simulink model "mesaparasimulink2"  (R2017a)
settings: Solver=ode3  StartTime=0.0  StopTime=3*1.256637  FixedStep=5e-3  RelTol=1e-3
values from neighbouring files (symbols this model uses):
  L1 = L1s(L1i)    [Resolver.m]    (also in calculodepar.m = L1/100)
  L2 = L2s(L2k)    [Resolver.m]    (also in calculodepar.m = L2/100)
  m = 6    [calculodepar.m]
  N = m*g - ten*sin(beta)    [calculodepar.m]    (also in main.m = 360; maindinamica.m = 360)
undefined symbols (not defined in the file or in its folder): bloque, bloque1, mesaparasimulink, pasador, RootGround, RootPart
libraries: mblibv1 x26, simulink x2
settings Model: Creator=angel  LastModifiedBy=angel
settings SimMechanicsCC: VisOnUpdateDiagram=on  VisDuringSimulation=on

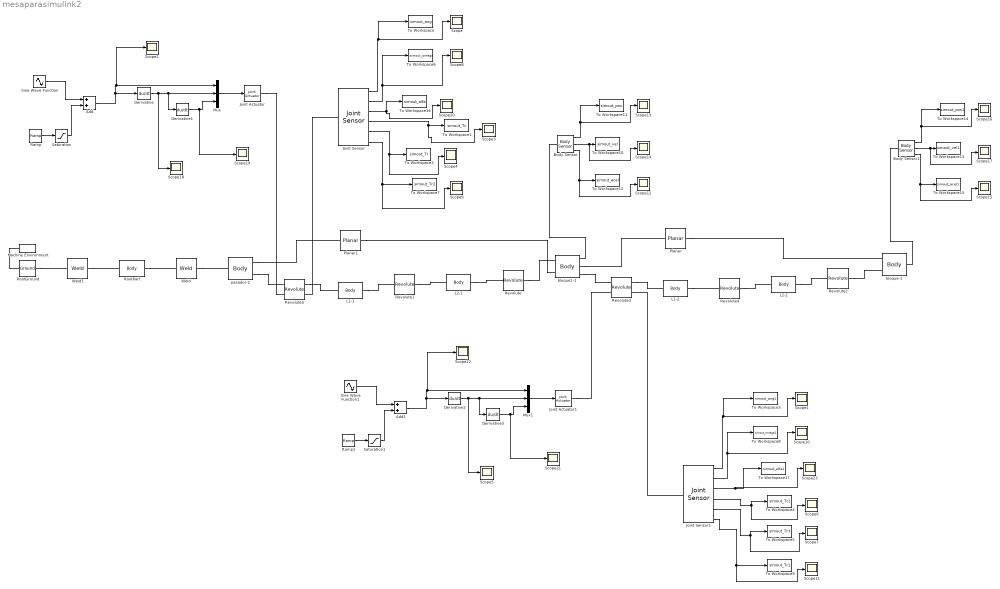
== system mesaparasimulink2 ==
  Add : Sum
  Add1 : Sum
  Body Sensor : mblibv1/Sensors &  Actuators/Body Sensor  UpdateFromCAD=off  PhysicalDomain=Mechanical  PortType=blob  Muxed=off  Pose=off  Angle=on  AngleUnits=deg  ArcVelocity=off  ArcVelocityUnits=deg/s  ArcAcceleration=off  ArcAccelerationUnits=deg/s^2  CoordPosition=on  CoordPositionUnits=cm  Velocity=on  VelocityUnits=cm/s  Acceleration=on  AccelerationUnits=cm/s^2  Quaternion=on  QuaternionDT=off  QuaternionDDT=off  QuaternionUnits=off  OutputVector=[1]  ActiveIO=on  Width=9  DialogClass=MechanicalSensorBlock  ReferenceFrame=Absolute (World)
      settings: SourceProductName=Simscape Multibody  SourceProductBaseCode=MS
  Body Sensor1 : mblibv1/Sensors &  Actuators/Body Sensor  UpdateFromCAD=off  PhysicalDomain=Mechanical  PortType=blob  Muxed=off  Pose=off  Angle=on  AngleUnits=deg  ArcVelocity=off  ArcVelocityUnits=deg/s  ArcAcceleration=off  ArcAccelerationUnits=deg/s^2  CoordPosition=on  CoordPositionUnits=cm  Velocity=on  VelocityUnits=cm/s  Acceleration=on  AccelerationUnits=cm/s^2  Quaternion=on  QuaternionDT=off  QuaternionDDT=off  QuaternionUnits=off  OutputVector=[1]  ActiveIO=on  Width=9  DialogClass=MechanicalSensorBlock  ReferenceFrame=Absolute (World)
      settings: SourceProductName=Simscape Multibody  SourceProductBaseCode=MS
  Derivative{,1..3} (4 alike) : Derivative  CoefficientInTFapproximation=1000
  Joint Actuator : mblibv1/Sensors &  Actuators/Joint Actuator  UpdateFromCAD=off  PhysicalDomain=Mechanical  PortType=blob  ActuationStyle=Motion  AngleUnits=deg  ArcVelocityUnits=deg/s  ArcAccelerationUnits=deg/s^2  CoordPositionUnits=m  VelocityUnits=m/s  AccelerationUnits=m/s^2  ForceUnits=N  TorqueUnits=N*m  ActiveIO=on  Width=3  DialogClass=MechanicalActuatorBlock  Primitive=R1  ReferenceFrame=Absolute (World)
      settings: SourceProductName=Simscape Multibody  SourceProductBaseCode=MS
  Joint Actuator1 : mblibv1/Sensors &  Actuators/Joint Actuator  UpdateFromCAD=off  PhysicalDomain=Mechanical  PortType=blob  ActuationStyle=Motion  AngleUnits=deg  ArcVelocityUnits=deg/s  ArcAccelerationUnits=deg/s^2  CoordPositionUnits=m  VelocityUnits=m/s  AccelerationUnits=m/s^2  ForceUnits=N  TorqueUnits=N*m  ActiveIO=on  Width=3  DialogClass=MechanicalActuatorBlock  Primitive=R1  ReferenceFrame=Absolute (World)
      settings: SourceProductName=Simscape Multibody  SourceProductBaseCode=MS
  Joint Sensor : mblibv1/Sensors &  Actuators/Joint Sensor  UpdateFromCAD=off  PhysicalDomain=Mechanical  PortType=blob  Muxed=off  Pose=off  Angle=on  AngleUnits=deg  ArcVelocity=on  ArcVelocityUnits=deg/s  ArcAcceleration=on  ArcAccelerationUnits=deg/s^2  CoordPosition=on  CoordPositionUnits=m  Velocity=off  VelocityUnits=m/s  Acceleration=off  AccelerationUnits=m/s^2  Quaternion=on  QuaternionDT=off  QuaternionDDT=off  QuaternionUnits=off  OutputVector=[1]  ActiveIO=on  Width=10  DialogClass=MechanicalSensorBlock  Primitive=R1  Force=off  ForceUnits=N  Torque=on  TorqueUnits=N*m  ReferenceFrame=Absolute (World)  ReactionSensedSide=Base  ReactionReferenceFrame=Absolute (World)  ReactionForce=on  ReactionForceUnits=N  ReactionMoment=on  ReactionMomentUnits=N*m
      settings: SourceProductName=Simscape Multibody  SourceProductBaseCode=MS
  Joint Sensor1 : mblibv1/Sensors &  Actuators/Joint Sensor  UpdateFromCAD=off  PhysicalDomain=Mechanical  PortType=blob  Muxed=off  Pose=off  Angle=on  AngleUnits=deg  ArcVelocity=on  ArcVelocityUnits=deg/s  ArcAcceleration=on  ArcAccelerationUnits=deg/s^2  CoordPosition=on  CoordPositionUnits=m  Velocity=off  VelocityUnits=m/s  Acceleration=off  AccelerationUnits=m/s^2  Quaternion=on  QuaternionDT=off  QuaternionDDT=off  QuaternionUnits=off  OutputVector=[1]  ActiveIO=on  Width=10  DialogClass=MechanicalSensorBlock  Primitive=R1  Force=off  ForceUnits=N  Torque=on  TorqueUnits=N*m  ReferenceFrame=Absolute (World)  ReactionSensedSide=Base  ReactionReferenceFrame=Absolute (World)  ReactionForce=on  ReactionForceUnits=N  ReactionMoment=on  ReactionMomentUnits=N*m
      settings: SourceProductName=Simscape Multibody  SourceProductBaseCode=MS
  L1-1 : mblibv1/Bodies/Body  LConnTagsString=CS3  RConnTagsString=CS2  UpdateFromCAD=on  PMImportedID=L1-1  DialogClass=MechanicalBodyBlock  Mass=0.00593014  MassUnits=kg  InertiaUnits=kg*m^2  Inertia=[1.04021e-06,0,0;0,1.07865e-06,0;0,0,6.31529e-08]  Shape=Cylinder  ShapeDims=[1 1]  ShapeUnits=m  ShapeUse=false  Density=1  DensityUnits=kg/m^3  DensityUse=false  GraphicsMode=GFXFILE  GraphicsFileName=mesaparasimulink - L1-1.STL  BodyColorSelMode=COLORPALETTE  BodyColor=[0.898039;0.917647;0.929412]  AttachedToCS=CS1  CG=Right$CG$[1.18183e-05 0.00118407 0.0299918]$WORLD$WORLD$m$[-0.999589 0 0.0286521;0 1 0;-0.0286521 0 -0.999589]$3x3 Transform$rad$WORLD$false$L1-1::CG(AUTOGEN)  WorkingFrames=Right$CS1$[0.00058486 -0.00131593 0.01]$WORLD$WORLD$m$[-0.999589 0 0.0286521;0 1 0;-0.0286521 0 -0.999589]$3x3 Transform$rad$WORLD$false$L1-1::CS1(AUTOGEN)#Right$CS2$[-0.000561223 0.00368407 0.0499836]$WORLD$WORLD$m$[1 0 0;0 1 0;0 0 1]$3x3 Transform$rad$WORLD$true$L1-1:-:L2-1::L1-1(AUTOGEN)#Left$CS3$[0.00058486 0.00368407 0.01]$WORLD$WORLD$m$[1 0 0;0 1 0;0 0 1]$3x3 Transform$rad$WORLD$true$L1-1:-:pasador-1::L1-1(AUTOGEN)  CGPos=[1.18183e-05 0.00118407 0.0299918]  CGRot=[-0.999589 0 0.0286521;0 1 0;-0.0286521 0 -0.999589]  CS0Pos=[]  CS0Rot=[]  CS1Pos=[0.00058486 -0.00131593 0.01]  CS1Rot=[-0.999589 0 0.0286521;0 1 0;-0.0286521 0 -0.999589]  CS2Pos=[-0.000561223 0.00368407 0.0499836]  CS2Rot=[1 0 0;0 1 0;0 0 1]  CS3Pos=[0.00058486 0.00368407 0.01]  CS3Rot=[1 0 0;0 1 0;0 0 1]  CS4Pos=[]  CS4Rot=[]  CS5Pos=[]  CS5Rot=[]  CS6Pos=[]  CS6Rot=[]  CS7Pos=[]  CS7Rot=[]  CS8Pos=[]  CS8Rot=[]  CS9Pos=[]  CS9Rot=[]  CS10Pos=[]  CS10Rot=[]  CS11Pos=[]  CS11Rot=[]  CS12Pos=[]  CS12Rot=[]  CS13Pos=[]  CS13Rot=[]  CS14Pos=[]  CS14Rot=[]  CS15Pos=[]  CS15Rot=[]  CS16Pos=[]  CS16Rot=[]  CS17Pos=[]  CS17Rot=[]  CS18Pos=[]  CS18Rot=[]  CS19Pos=[]  CS19Rot=[]  CS20Pos=[]  CS20Rot=[]
      settings: SourceProductName=Simscape Multibody  SourceProductBaseCode=MS
  L1-2 : mblibv1/Bodies/Body  LConnTagsString=CS2  RConnTagsString=CS3  UpdateFromCAD=on  PMImportedID=L1-2  DialogClass=MechanicalBodyBlock  Mass=0.00593014  MassUnits=kg  InertiaUnits=kg*m^2  Inertia=[1.04021e-06,0,0;0,1.07865e-06,0;0,0,6.31529e-08]  Shape=Cylinder  ShapeDims=[1 1]  ShapeUnits=m  ShapeUse=false  Density=1  DensityUnits=kg/m^3  DensityUse=false  GraphicsMode=GFXFILE  GraphicsFileName=mesaparasimulink - L1-2.STL  BodyColorSelMode=COLORPALETTE  BodyColor=[0.898039;0.917647;0.929412]  AttachedToCS=CS1  CG=Right$CG$[0.23557 0.0339841 -0.180783]$WORLD$WORLD$m$[0.0387738 0 -0.999248;0 1 0;0.999248 0 0.0387738]$3x3 Transform$rad$WORLD$false$L1-2::CG(AUTOGEN)  WorkingFrames=Right$CS1$[0.215585 0.0314841 -0.180007]$WORLD$WORLD$m$[0.0387738 0 -0.999248;0 1 0;0.999248 0 0.0387738]$3x3 Transform$rad$WORLD$false$L1-2::CS1(AUTOGEN)#Left$CS2$[0.215585 0.0364841 -0.180007]$WORLD$WORLD$m$[1 0 0;0 1 0;0 0 1]$3x3 Transform$rad$WORLD$true$L1-2:-:bloque1-1::L1-2(AUTOGEN)#Right$CS3$[0.255555 0.0364841 -0.181558]$WORLD$WORLD$m$[1 0 0;0 1 0;0 0 1]$3x3 Transform$rad$WORLD$true$L1-2:-:L2-2::L1-2(AUTOGEN)  CGPos=[0.23557 0.0339841 -0.180783]  CGRot=[0.0387738 0 -0.999248;0 1 0;0.999248 0 0.0387738]  CS0Pos=[]  CS0Rot=[]  CS1Pos=[0.215585 0.0314841 -0.180007]  CS1Rot=[0.0387738 0 -0.999248;0 1 0;0.999248 0 0.0387738]  CS2Pos=[0.215585 0.0364841 -0.180007]  CS2Rot=[1 0 0;0 1 0;0 0 1]  CS3Pos=[0.255555 0.0364841 -0.181558]  CS3Rot=[1 0 0;0 1 0;0 0 1]  CS4Pos=[]  CS4Rot=[]  CS5Pos=[]  CS5Rot=[]  CS6Pos=[]  CS6Rot=[]  CS7Pos=[]  CS7Rot=[]  CS8Pos=[]  CS8Rot=[]  CS9Pos=[]  CS9Rot=[]  CS10Pos=[]  CS10Rot=[]  CS11Pos=[]  CS11Rot=[]  CS12Pos=[]  CS12Rot=[]  CS13Pos=[]  CS13Rot=[]  CS14Pos=[]  CS14Rot=[]  CS15Pos=[]  CS15Rot=[]  CS16Pos=[]  CS16Rot=[]  CS17Pos=[]  CS17Rot=[]  CS18Pos=[]  CS18Rot=[]  CS19Pos=[]  CS19Rot=[]  CS20Pos=[]  CS20Rot=[]
      settings: SourceProductName=Simscape Multibody  SourceProductBaseCode=MS
  L2-1 : mblibv1/Bodies/Body  LConnTagsString=CS3  RConnTagsString=CS2  UpdateFromCAD=on  PMImportedID=L2-1  DialogClass=MechanicalBodyBlock  Mass=0.00998014  MassUnits=kg  InertiaUnits=kg*m^2  Inertia=[4.69227e-06,0,0;0,4.75602e-06,0;0,0,1.0534e-07]  Shape=Cylinder  ShapeDims=[1 1]  ShapeUnits=m  ShapeUse=false  Density=1  DensityUnits=kg/m^3  DensityUse=false  GraphicsMode=GFXFILE  GraphicsFileName=mesaparasimulink - L2-1.STL  BodyColorSelMode=COLORPALETTE  BodyColor=[0.898039;0.917647;0.929412]  AttachedToCS=CS1  CG=Right$CG$[1.18183e-05 0.00618407 0.0149883]$WORLD$WORLD$m$[0.999866 0 -0.0163726;0 1 0;0.0163726 0 0.999866]$3x3 Transform$rad$WORLD$false$L2-1::CG(AUTOGEN)  WorkingFrames=Right$CS1$[-0.000561223 0.00368407 0.0499836]$WORLD$WORLD$m$[0.999866 0 -0.0163726;0 1 0;0.0163726 0 0.999866]$3x3 Transform$rad$WORLD$false$L2-1::CS1(AUTOGEN)#Right$CS2$[0.00058486 0.00368407 -0.020007]$WORLD$WORLD$m$[1 0 0;0 1 0;0 0 1]$3x3 Transform$rad$WORLD$true$L2-1:-:bloque1-1::L2-1(AUTOGEN)#Left$CS3$[-0.000561223 0.00368407 0.0499836]$WORLD$WORLD$m$[1 0 0;0 1 0;0 0 1]$3x3 Transform$rad$WORLD$true$L1-1:-:L2-1::L2-1(AUTOGEN)  CGPos=[1.18183e-05 0.00618407 0.0149883]  CGRot=[0.999866 0 -0.0163726;0 1 0;0.0163726 0 0.999866]  CS0Pos=[]  CS0Rot=[]  CS1Pos=[-0.000561223 0.00368407 0.0499836]  CS1Rot=[0.999866 0 -0.0163726;0 1 0;0.0163726 0 0.999866]  CS2Pos=[0.00058486 0.00368407 -0.020007]  CS2Rot=[1 0 0;0 1 0;0 0 1]  CS3Pos=[-0.000561223 0.00368407 0.0499836]  CS3Rot=[1 0 0;0 1 0;0 0 1]  CS4Pos=[]  CS4Rot=[]  CS5Pos=[]  CS5Rot=[]  CS6Pos=[]  CS6Rot=[]  CS7Pos=[]  CS7Rot=[]  CS8Pos=[]  CS8Rot=[]  CS9Pos=[]  CS9Rot=[]  CS10Pos=[]  CS10Rot=[]  CS11Pos=[]  CS11Rot=[]  CS12Pos=[]  CS12Rot=[]  CS13Pos=[]  CS13Rot=[]  CS14Pos=[]  CS14Rot=[]  CS15Pos=[]  CS15Rot=[]  CS16Pos=[]  CS16Rot=[]  CS17Pos=[]  CS17Rot=[]  CS18Pos=[]  CS18Rot=[]  CS19Pos=[]  CS19Rot=[]  CS20Pos=[]  CS20Rot=[]
      settings: SourceProductName=Simscape Multibody  SourceProductBaseCode=MS
  L2-2 : mblibv1/Bodies/Body  LConnTagsString=CS3  RConnTagsString=CS2  UpdateFromCAD=on  PMImportedID=L2-2  DialogClass=MechanicalBodyBlock  Mass=0.00998014  MassUnits=kg  InertiaUnits=kg*m^2  Inertia=[4.69227e-06,0,0;0,4.75602e-06,0;0,0,1.0534e-07]  Shape=Cylinder  ShapeDims=[1 1]  ShapeUnits=m  ShapeUse=false  Density=1  DensityUnits=kg/m^3  DensityUse=false  GraphicsMode=GFXFILE  GraphicsFileName=mesaparasimulink - L2-2.STL  BodyColorSelMode=COLORPALETTE  BodyColor=[0.898039;0.917647;0.929412]  AttachedToCS=CS1  CG=Right$CG$[0.220563 0.0389841 -0.180783]$WORLD$WORLD$m$[-0.0221564 0 0.999755;0 1 0;-0.999755 0 -0.0221564]$3x3 Transform$rad$WORLD$false$L2-2::CG(AUTOGEN)  WorkingFrames=Right$CS1$[0.255555 0.0364841 -0.181558]$WORLD$WORLD$m$[-0.0221564 0 0.999755;0 1 0;-0.999755 0 -0.0221564]$3x3 Transform$rad$WORLD$false$L2-2::CS1(AUTOGEN)#Right$CS2$[0.185572 0.0414841 -0.180007]$WORLD$WORLD$m$[1 0 0;0 1 0;0 0 1]$3x3 Transform$rad$WORLD$true$L2-2:-:bloque-1::L2-2(AUTOGEN)#Left$CS3$[0.255555 0.0364841 -0.181558]$WORLD$WORLD$m$[1 0 0;0 1 0;0 0 1]$3x3 Transform$rad$WORLD$true$L1-2:-:L2-2::L2-2(AUTOGEN)  CGPos=[0.220563 0.0389841 -0.180783]  CGRot=[-0.0221564 0 0.999755;0 1 0;-0.999755 0 -0.0221564]  CS0Pos=[]  CS0Rot=[]  CS1Pos=[0.255555 0.0364841 -0.181558]  CS1Rot=[-0.0221564 0 0.999755;0 1 0;-0.999755 0 -0.0221564]  CS2Pos=[0.185572 0.0414841 -0.180007]  CS2Rot=[1 0 0;0 1 0;0 0 1]  CS3Pos=[0.255555 0.0364841 -0.181558]  CS3Rot=[1 0 0;0 1 0;0 0 1]  CS4Pos=[]  CS4Rot=[]  CS5Pos=[]  CS5Rot=[]  CS6Pos=[]  CS6Rot=[]  CS7Pos=[]  CS7Rot=[]  CS8Pos=[]  CS8Rot=[]  CS9Pos=[]  CS9Rot=[]  CS10Pos=[]  CS10Rot=[]  CS11Pos=[]  CS11Rot=[]  CS12Pos=[]  CS12Rot=[]  CS13Pos=[]  CS13Rot=[]  CS14Pos=[]  CS14Rot=[]  CS15Pos=[]  CS15Rot=[]  CS16Pos=[]  CS16Rot=[]  CS17Pos=[]  CS17Rot=[]  CS18Pos=[]  CS18Rot=[]  CS19Pos=[]  CS19Rot=[]  CS20Pos=[]  CS20Rot=[]
      settings: SourceProductName=Simscape Multibody  SourceProductBaseCode=MS
  Machine Environment : mblibv1/Bodies/Machine Environment  PortType=env  PhysicalDomain=Mechanical  DialogTemplateClass=MECH.MachineEnvironment  SyncWhenCopied=off  Gravity=[0 -9.81 0]  GravityUnits=m/s^2  GravityAsSignal=off  Dimensionality=Auto-detect  AnalysisType=Forward dynamics  LinearAssemblyTolerance=1e-3  LinearAssemblyToleranceUnits=m  AngularAssemblyTolerance=1e-3  AngularAssemblyToleranceUnits=rad  ConstraintSolverType=Stabilizing  ConstraintRelTolerance=1e-4  ConstraintAbsTolerance=1e-4  UseRobustSingularityHandling=off  RedundancyAnalysisToleranceType=Automatically select tolerance  RedundancyAnalysisTolerance=1e-14  StatePerturbationType=Fixed  PerturbationSize=1e-5  VisualizeMachine=on  BodyVisualizationType=Use model default body geometries  BodyColorSelMode=Use model default  DefaultBodyColor=[1 0 0]
      settings: SourceProductName=Simscape Multibody  SourceProductBaseCode=MS
  Mux : Mux  Inputs=3
  Mux1 : Mux  Inputs=3
  Planar : mblibv1/Joints/Planar  LConnTagsString=__newl0  RConnTagsString=__newr0  UpdateFromCAD=on  PMImportedID=bloque-1:-:bloque1-1  NumSAPorts=0  CutJoint=off  MarkAsCut=off  Primitives=prismatic_prismatic  PrimitiveProps=P1$WORLD$[1,0,0]$prismatic#P2$WORLD$[0,-1,0]$prismatic#R1$WORLD$[0,0,1]$revolute  DialogClass=JointBlock  P1Axis=[1,0,0]  P2Axis=[0,-1,0]  R1Axis=[0,0,1]
      settings: SourceProductName=Simscape Multibody  SourceProductBaseCode=MS
  Planar1 : mblibv1/Joints/Planar  LConnTagsString=__newl0  RConnTagsString=__newr0  UpdateFromCAD=on  PMImportedID=bloque1-1:-:pasador-1  NumSAPorts=0  CutJoint=off  MarkAsCut=off  Primitives=prismatic_prismatic  PrimitiveProps=P1$WORLD$[0,1,0]$prismatic#P2$WORLD$[0,0,1]$prismatic#R1$WORLD$[-1,0,0]$revolute  DialogClass=JointBlock  P1Axis=[0,1,0]  P2Axis=[0,0,1]  R1Axis=[-1,0,0]
      settings: SourceProductName=Simscape Multibody  SourceProductBaseCode=MS
  Ramp : simulink/Sources/Ramp  slope=2000  start=0  X0=0
  Ramp1 : simulink/Sources/Ramp  slope=2000  start=0  X0=0
  Revolute : mblibv1/Joints/Revolute  LConnTagsString=__newl0  RConnTagsString=__newr0  UpdateFromCAD=on  PMImportedID=L2-1:-:bloque1-1  NumSAPorts=0  CutJoint=off  MarkAsCut=off  Primitives=prismatic  PrimitiveProps=R1$WORLD$[0,-1,0]$revolute  DialogClass=JointBlock  R1Axis=[0,-1,0]
      settings: SourceProductName=Simscape Multibody  SourceProductBaseCode=MS
  Revolute1 : mblibv1/Joints/Revolute  LConnTagsString=__newl0  RConnTagsString=__newr0  UpdateFromCAD=on  PMImportedID=L1-1:-:L2-1  NumSAPorts=0  CutJoint=off  MarkAsCut=off  Primitives=prismatic  PrimitiveProps=R1$WORLD$[0,1,0]$revolute  DialogClass=JointBlock  R1Axis=[0,1,0]
      settings: SourceProductName=Simscape Multibody  SourceProductBaseCode=MS
  Revolute2 : mblibv1/Joints/Revolute  LConnTagsString=__newl0  RConnTagsString=__newr0  UpdateFromCAD=on  PMImportedID=L2-2:-:bloque-1  NumSAPorts=0  CutJoint=off  MarkAsCut=off  Primitives=prismatic  PrimitiveProps=R1$WORLD$[0,-1,0]$revolute  DialogClass=JointBlock  R1Axis=[0,-1,0]
      settings: SourceProductName=Simscape Multibody  SourceProductBaseCode=MS
  Revolute3 : mblibv1/Joints/Revolute  LConnTagsString=__newl0|SA1  RConnTagsString=__newr0|SA1  UpdateFromCAD=on  PMImportedID=L1-2:-:bloque1-1  NumSAPorts=2  CutJoint=off  MarkAsCut=off  Primitives=prismatic  PrimitiveProps=R1$World$[0,-1,0]$revolute  DialogClass=JointBlock  R1Axis=[0,-1,0]
      settings: SourceProductName=Simscape Multibody  SourceProductBaseCode=MS
  Revolute4 : mblibv1/Joints/Revolute  LConnTagsString=__newl0  RConnTagsString=__newr0  UpdateFromCAD=on  PMImportedID=L1-2:-:L2-2  NumSAPorts=0  CutJoint=off  MarkAsCut=off  Primitives=prismatic  PrimitiveProps=R1$WORLD$[0,1,0]$revolute  DialogClass=JointBlock  R1Axis=[0,1,0]
      settings: SourceProductName=Simscape Multibody  SourceProductBaseCode=MS
  Revolute5 : mblibv1/Joints/Revolute  LConnTagsString=__newl0|SA1  RConnTagsString=__newr0|SA1  UpdateFromCAD=on  PMImportedID=L1-1:-:pasador-1  NumSAPorts=2  CutJoint=off  MarkAsCut=off  Primitives=prismatic  PrimitiveProps=R1$World$[0,-1,0]$revolute  DialogClass=JointBlock  R1Axis=[0,-1,0]
      settings: SourceProductName=Simscape Multibody  SourceProductBaseCode=MS
  RootGround : mblibv1/Bodies/Ground  UpdateFromCAD=on  PMImportedID=RootGround  LeftPortType=env  RightPortType=workingframe  PhysicalDomain=Mechanical  DialogClass=GroundBlock  CoordPosition=[0.0320269,0.0170753,-0.177764]  CoordPositionUnits=m  StateVectorMgrId=12  MachineId=[13 0]  ShowEnvPort=on  ParameterChecksum=[852557314, 1956477998, 3151099103, 2810695975]  TopologyChecksum=[577523957, 3827055526, 3732085488, 4080315241]
      settings: SourceProductName=Simscape Multibody  SourceProductBaseCode=MS
  RootPart : mblibv1/Bodies/Body  LConnTagsString=CS3  RConnTagsString=CS2  UpdateFromCAD=on  PMImportedID=mesaparasimulink/RootPart  DialogClass=MechanicalBodyBlock  Mass=0  MassUnits=kg  InertiaUnits=kg*m^2  Inertia=[0,0,0;0,0,0;0,0,0]  Shape=Cylinder  ShapeDims=[1 1]  ShapeUnits=m  ShapeUse=false  Density=1  DensityUnits=kg/m^3  DensityUse=false  GraphicsMode=MACHINE_DEFAULT  BodyColorSelMode=MACHINE_DEFAULT  BodyColor=[1;0;0]  AttachedToCS=CS1  CG=Right$CG$[0.0320269 0.0170753 -0.177764]$WORLD$WORLD$m$[1 0 0;0 1 0;0 0 1]$3x3 Transform$rad$WORLD$false$mesaparasimulink/RootPart::CG(AUTOGEN)  WorkingFrames=Right$CS1$[0 0 0]$WORLD$WORLD$m$[1 0 0;0 1 0;0 0 1]$3x3 Transform$rad$WORLD$false$mesaparasimulink/RootPart::CS1(AUTOGEN)#Right$CS2$[0.0153072 0.00615805 -0.0448119]$WORLD$WORLD$m$[1 0 0;0 1 0;0 0 1]$3x3 Transform$rad$WORLD$true$mesaparasimulink/RootPart:-:pasador-1::mesaparasimulink/RootPart(AUTOGEN)#Left$CS3$[0.0320269 0.0170753 -0.177764]$WORLD$WORLD$m$[1 0 0;0 1 0;0 0 1]$3x3 Transform$rad$WORLD$true$RootGround:-:mesaparasimulink/RootPart::mesaparasimulink/RootPart(AUTOGEN)  CGPos=[0.0320269 0.0170753 -0.177764]  CGRot=[1 0 0;0 1 0;0 0 1]  CS0Pos=[]  CS0Rot=[]  CS1Pos=[0 0 0]  CS1Rot=[1 0 0;0 1 0;0 0 1]  CS2Pos=[0.0153072 0.00615805 -0.0448119]  CS2Rot=[1 0 0;0 1 0;0 0 1]  CS3Pos=[0.0320269 0.0170753 -0.177764]  CS3Rot=[1 0 0;0 1 0;0 0 1]  CS4Pos=[]  CS4Rot=[]  CS5Pos=[]  CS5Rot=[]  CS6Pos=[]  CS6Rot=[]  CS7Pos=[]  CS7Rot=[]  CS8Pos=[]  CS8Rot=[]  CS9Pos=[]  CS9Rot=[]  CS10Pos=[]  CS10Rot=[]  CS11Pos=[]  CS11Rot=[]  CS12Pos=[]  CS12Rot=[]  CS13Pos=[]  CS13Rot=[]  CS14Pos=[]  CS14Rot=[]  CS15Pos=[]  CS15Rot=[]  CS16Pos=[]  CS16Rot=[]  CS17Pos=[]  CS17Rot=[]  CS18Pos=[]  CS18Rot=[]  CS19Pos=[]  CS19Rot=[]  CS20Pos=[]  CS20Rot=[]
      settings: SourceProductName=Simscape Multibody  SourceProductBaseCode=MS
  Saturation : Saturate  UpperLimit=245
  Saturation1 : Saturate  UpperLimit=245
  Scope{,1..23} (24 alike) : Scope
  Sine Wave Function : Sin  Amplitude=14.455*1  Frequency=2*pi*5  SampleTime=0
  Sine Wave Function1 : Sin  Amplitude=14.455*1  Frequency=2*pi*5  SampleTime=0
  To Workspace : ToWorkspace  VariableName=simout_ang  SaveFormat=Structure With Time  SampleTime=-1
  To Workspace1 : ToWorkspace  VariableName=simout_Tc  SaveFormat=Structure With Time  SampleTime=-1
  To Workspace10 : ToWorkspace  VariableName=simout_vel  SaveFormat=Structure With Time  SampleTime=-1
  To Workspace11 : ToWorkspace  VariableName=simout_pos  SaveFormat=Structure With Time  SampleTime=-1
  To Workspace12 : ToWorkspace  VariableName=simout_acel  SaveFormat=Structure With Time  SampleTime=-1
  To Workspace13 : ToWorkspace  VariableName=simout_vel1  SaveFormat=Structure With Time  SampleTime=-1
  To Workspace14 : ToWorkspace  VariableName=simout_pos1  SaveFormat=Structure With Time  SampleTime=-1
  To Workspace15 : ToWorkspace  VariableName=simout_acel1  SaveFormat=Structure With Time  SampleTime=-1
  To Workspace16 : ToWorkspace  VariableName=simout_alfa  SaveFormat=Structure With Time  SampleTime=-1
  To Workspace17 : ToWorkspace  VariableName=simout_alfa1  SaveFormat=Structure With Time  SampleTime=-1
  To Workspace2 : ToWorkspace  VariableName=simout_Tr  SaveFormat=Structure With Time  SampleTime=-1
  To Workspace3 : ToWorkspace  VariableName=simout_ang1  SaveFormat=Structure With Time  SampleTime=-1
  To Workspace4 : ToWorkspace  VariableName=simout_Tc1  SaveFormat=Structure With Time  SampleTime=-1
  To Workspace5 : ToWorkspace  VariableName=simout_Tr3  SaveFormat=Structure With Time  SampleTime=-1
  To Workspace6 : ToWorkspace  VariableName=simout_omega  SaveFormat=Structure With Time  SampleTime=-1
  To Workspace7 : ToWorkspace  VariableName=simout_Tr2  SaveFormat=Structure With Time  SampleTime=-1
  To Workspace8 : ToWorkspace  VariableName=simout_omega1  SaveFormat=Structure With Time  SampleTime=-1
  To Workspace9 : ToWorkspace  VariableName=simout_Tr1  SaveFormat=Structure With Time  SampleTime=-1
  Weld : mblibv1/Joints/Weld  LConnTagsString=__newl0  RConnTagsString=__newr0  UpdateFromCAD=on  PMImportedID=mesaparasimulink/RootPart:-:pasador-1  NumSAPorts=0  CutJoint=off  MarkAsCut=off  Primitives=weld  PrimitiveProps=W$WORLD$[0.57735,0.57735,0.57735]$weld  DialogClass=JointBlock  WAxis=[0.57735,0.57735,0.57735]
      settings: SourceProductName=Simscape Multibody  SourceProductBaseCode=MS
  Weld1 : mblibv1/Joints/Weld  LConnTagsString=__newl0  RConnTagsString=__newr0  UpdateFromCAD=on  PMImportedID=RootGround:-:mesaparasimulink/RootPart  NumSAPorts=0  CutJoint=off  MarkAsCut=off  Primitives=weld  PrimitiveProps=W$WORLD$[0.57735,0.57735,0.57735]$weld  DialogClass=JointBlock  WAxis=[0.57735,0.57735,0.57735]
      settings: SourceProductName=Simscape Multibody  SourceProductBaseCode=MS
  bloque-1 : mblibv1/Bodies/Body  LConnTagsString=CS2|CS3  RConnTagsString=CS1  UpdateFromCAD=on  PMImportedID=bloque-1  DialogClass=MechanicalBodyBlock  Mass=0.678513  MassUnits=kg  InertiaUnits=kg*m^2  Inertia=[0.0082438,0,0;0,0.0168493,0;0,0,0.00868909]  Shape=Cylinder  ShapeDims=[1 1]  ShapeUnits=m  ShapeUse=false  Density=1  DensityUnits=kg/m^3  DensityUse=false  GraphicsMode=GFXFILE  GraphicsFileName=mesaparasimulink - bloque-1.STL  BodyColorSelMode=COLORPALETTE  BodyColor=[0.64706 0.61961 0.58823]  AttachedToCS=CS1  CG=Right$CG$[0.0298846 0.0389841 -0.180007]$WORLD$WORLD$m$[1 0 0;0 1 0;0 0 1]$3x3 Transform$rad$WORLD$false$bloque-1::CG(AUTOGEN)  WorkingFrames=Right$CS1$[0.025572 0.0389841 -0.180007]$WORLD$WORLD$m$[1 0 0;0 1 0;0 0 1]$3x3 Transform$rad$WORLD$true$bloque-1::CS1(AUTOGEN)#Left$CS2$[0.129445 0.0614841 -0.185007]$WORLD$WORLD$m$[1 0 0;0 1 0;0 0 1]$3x3 Transform$rad$WORLD$true$bloque-1:-:bloque1-1::bloque-1(AUTOGEN)#Left$CS3$[0.185572 0.0414841 -0.180007]$WORLD$WORLD$m$[1 0 0;0 1 0;0 0 1]$3x3 Transform$rad$WORLD$true$L2-2:-:bloque-1::bloque-1(AUTOGEN)  CGPos=[0.0298846 0.0389841 -0.180007]  CGRot=[1 0 0;0 1 0;0 0 1]  CS0Pos=[]  CS0Rot=[]  CS1Pos=[0.025572 0.0389841 -0.180007]  CS1Rot=[1 0 0;0 1 0;0 0 1]  CS2Pos=[0.129445 0.0614841 -0.185007]  CS2Rot=[1 0 0;0 1 0;0 0 1]  CS3Pos=[0.185572 0.0414841 -0.180007]  CS3Rot=[1 0 0;0 1 0;0 0 1]  CS4Pos=[]  CS4Rot=[]  CS5Pos=[]  CS5Rot=[]  CS6Pos=[]  CS6Rot=[]  CS7Pos=[]  CS7Rot=[]  CS8Pos=[]  CS8Rot=[]  CS9Pos=[]  CS9Rot=[]  CS10Pos=[]  CS10Rot=[]  CS11Pos=[]  CS11Rot=[]  CS12Pos=[]  CS12Rot=[]  CS13Pos=[]  CS13Rot=[]  CS14Pos=[]  CS14Rot=[]  CS15Pos=[]  CS15Rot=[]  CS16Pos=[]  CS16Rot=[]  CS17Pos=[]  CS17Rot=[]  CS18Pos=[]  CS18Rot=[]  CS19Pos=[]  CS19Rot=[]  CS20Pos=[]  CS20Rot=[]
      settings: SourceProductName=Simscape Multibody  SourceProductBaseCode=MS
  bloque1-1 : mblibv1/Bodies/Body  LConnTagsString=CS2|CS4  RConnTagsString=CS1|CS3|CS5  UpdateFromCAD=on  PMImportedID=bloque1-1  DialogClass=MechanicalBodyBlock  Mass=1.56446  MassUnits=kg  InertiaUnits=kg*m^2  Inertia=[0.0197353,-0.000140347,-0.00048114;-0.000140347,0.0283788,-0.00130115;-0.00048114,-0.00130115,0.00966506]  Shape=Cylinder  ShapeDims=[1 1]  ShapeUnits=m  ShapeUse=false  Density=1  DensityUnits=kg/m^3  DensityUse=false  GraphicsMode=GFXFILE  GraphicsFileName=mesaparasimulink - bloque1-1.STL  BodyColorSelMode=COLORPALETTE  BodyColor=[0.64706 0.61961 0.58823]  AttachedToCS=CS1  CG=Right$CG$[0.0315251 0.0076415 -0.180509]$WORLD$WORLD$m$[0 0 1;0 1 0;-1 0 0]$3x3 Transform$rad$WORLD$false$bloque1-1::CG(AUTOGEN)  WorkingFrames=Right$CS1$[0.00058486 0.00618407 -0.180007]$WORLD$WORLD$m$[0 0 1;0 1 0;-1 0 0]$3x3 Transform$rad$WORLD$true$bloque1-1::CS1(AUTOGEN)#Left$CS2$[0.00058486 0.00368407 -0.020007]$WORLD$WORLD$m$[1 0 0;0 1 0;0 0 1]$3x3 Transform$rad$WORLD$true$L2-1:-:bloque1-1::bloque1-1(AUTOGEN)#Right$CS3$[0.129445 0.0614841 -0.185007]$WORLD$WORLD$m$[1 0 0;0 1 0;0 0 1]$3x3 Transform$rad$WORLD$true$bloque-1:-:bloque1-1::bloque1-1(AUTOGEN)#Left$CS4$[0.00558486 0.0186841 -0.0657822]$WORLD$WORLD$m$[1 0 0;0 1 0;0 0 1]$3x3 Transform$rad$WORLD$true$bloque1-1:-:pasador-1::bloque1-1(AUTOGEN)#Right$CS5$[0.215585 0.0364841 -0.180007]$WORLD$WORLD$m$[1 0 0;0 1 0;0 0 1]$3x3 Transform$rad$WORLD$true$L1-2:-:bloque1-1::bloque1-1(AUTOGEN)  CGPos=[0.0315251 0.0076415 -0.180509]  CGRot=[0 0 1;0 1 0;-1 0 0]  CS0Pos=[]  CS0Rot=[]  CS1Pos=[0.00058486 0.00618407 -0.180007]  CS1Rot=[0 0 1;0 1 0;-1 0 0]  CS2Pos=[0.00058486 0.00368407 -0.020007]  CS2Rot=[1 0 0;0 1 0;0 0 1]  CS3Pos=[0.129445 0.0614841 -0.185007]  CS3Rot=[1 0 0;0 1 0;0 0 1]  CS4Pos=[0.00558486 0.0186841 -0.0657822]  CS4Rot=[1 0 0;0 1 0;0 0 1]  CS5Pos=[0.215585 0.0364841 -0.180007]  CS5Rot=[1 0 0;0 1 0;0 0 1]  CS6Pos=[]  CS6Rot=[]  CS7Pos=[]  CS7Rot=[]  CS8Pos=[]  CS8Rot=[]  CS9Pos=[]  CS9Rot=[]  CS10Pos=[]  CS10Rot=[]  CS11Pos=[]  CS11Rot=[]  CS12Pos=[]  CS12Rot=[]  CS13Pos=[]  CS13Rot=[]  CS14Pos=[]  CS14Rot=[]  CS15Pos=[]  CS15Rot=[]  CS16Pos=[]  CS16Rot=[]  CS17Pos=[]  CS17Rot=[]  CS18Pos=[]  CS18Rot=[]  CS19Pos=[]  CS19Rot=[]  CS20Pos=[]  CS20Rot=[]
      settings: SourceProductName=Simscape Multibody  SourceProductBaseCode=MS
  pasador-1 : mblibv1/Bodies/Body  LConnTagsString=CS2  RConnTagsString=CS3|CS4  UpdateFromCAD=on  PMImportedID=pasador-1  DialogClass=MechanicalBodyBlock  Mass=0.0203797  MassUnits=kg  InertiaUnits=kg*m^2  Inertia=[4.19852e-06,-7.80496e-09,5.72392e-08;-7.80496e-09,3.79828e-06,2.90582e-08;5.72392e-08,2.90582e-08,1.72439e-06]  Shape=Cylinder  ShapeDims=[1 1]  ShapeUnits=m  ShapeUse=false  Density=1  DensityUnits=kg/m^3  DensityUse=false  GraphicsMode=GFXFILE  GraphicsFileName=mesaparasimulink - pasador-1.STL  BodyColorSelMode=COLORPALETTE  BodyColor=[0.792157;0.819608;0.933333]  AttachedToCS=CS1  CG=Right$CG$[0.0153072 0.00615805 -0.0448119]$WORLD$WORLD$m$[1 0 0;0 1 0;0 0 1]$3x3 Transform$rad$WORLD$false$pasador-1::CG(AUTOGEN)  WorkingFrames=Right$CS1$[0.00058486 -0.00631593 0.01]$WORLD$WORLD$m$[1 0 0;0 1 0;0 0 1]$3x3 Transform$rad$WORLD$false$pasador-1::CS1(AUTOGEN)#Left$CS2$[0.0153072 0.00615805 -0.0448119]$WORLD$WORLD$m$[1 0 0;0 1 0;0 0 1]$3x3 Transform$rad$WORLD$true$mesaparasimulink/RootPart:-:pasador-1::pasador-1(AUTOGEN)#Right$CS3$[0.00558486 0.0186841 -0.0657822]$WORLD$WORLD$m$[1 0 0;0 1 0;0 0 1]$3x3 Transform$rad$WORLD$true$bloque1-1:-:pasador-1::pasador-1(AUTOGEN)#Right$CS4$[0.00058486 0.00368407 0.01]$WORLD$WORLD$m$[1 0 0;0 1 0;0 0 1]$3x3 Transform$rad$WORLD$true$L1-1:-:pasador-1::pasador-1(AUTOGEN)  CGPos=[0.0153072 0.00615805 -0.0448119]  CGRot=[1 0 0;0 1 0;0 0 1]  CS0Pos=[]  CS0Rot=[]  CS1Pos=[0.00058486 -0.00631593 0.01]  CS1Rot=[1 0 0;0 1 0;0 0 1]  CS2Pos=[0.0153072 0.00615805 -0.0448119]  CS2Rot=[1 0 0;0 1 0;0 0 1]  CS3Pos=[0.00558486 0.0186841 -0.0657822]  CS3Rot=[1 0 0;0 1 0;0 0 1]  CS4Pos=[0.00058486 0.00368407 0.01]  CS4Rot=[1 0 0;0 1 0;0 0 1]  CS5Pos=[]  CS5Rot=[]  CS6Pos=[]  CS6Rot=[]  CS7Pos=[]  CS7Rot=[]  CS8Pos=[]  CS8Rot=[]  CS9Pos=[]  CS9Rot=[]  CS10Pos=[]  CS10Rot=[]  CS11Pos=[]  CS11Rot=[]  CS12Pos=[]  CS12Rot=[]  CS13Pos=[]  CS13Rot=[]  CS14Pos=[]  CS14Rot=[]  CS15Pos=[]  CS15Rot=[]  CS16Pos=[]  CS16Rot=[]  CS17Pos=[]  CS17Rot=[]  CS18Pos=[]  CS18Rot=[]  CS19Pos=[]  CS19Rot=[]  CS20Pos=[]  CS20Rot=[]
      settings: SourceProductName=Simscape Multibody  SourceProductBaseCode=MS
  wires:
  Derivative1/1 -> Scope19/1, Mux/3
  Derivative/1 -> Scope18/1, Derivative1/1, Mux/2
  Joint Sensor/4 -> Scope3/1, To Workspace1/1
  Joint Sensor/6 -> Scope9/1, To Workspace7/1
  Sine Wave Function/1 -> Add/1
  Joint Sensor/2 -> Scope8/1, To Workspace6/1
  Add/1 -> Scope2/1, Mux/1, Derivative/1
  Joint Sensor/1 -> Scope/1, To Workspace/1
  Mux/1 -> Joint Actuator/1
  Joint Sensor/5 -> Scope4/1, To Workspace2/1
  Joint Sensor/3 -> To Workspace16/1, Scope20/1
  Derivative3/1 -> Scope21/1, Mux1/3
  Sine Wave Function1/1 -> Add1/1
  Mux1/1 -> Joint Actuator1/1
  Joint Sensor1/5 -> To Workspace5/1, Scope7/1
  Joint Sensor1/2 -> Scope10/1, To Workspace8/1
  Add1/1 -> Scope22/1, Mux1/1, Derivative2/1
  Joint Sensor1/3 -> Scope23/1, To Workspace17/1
  Joint Sensor1/6 -> Scope11/1, To Workspace9/1
  Joint Sensor1/4 -> Scope6/1, To Workspace4/1
  Joint Sensor1/1 -> Scope1/1, To Workspace3/1
  Derivative2/1 -> Scope5/1, Derivative3/1, Mux1/2
  Body Sensor/1 -> To Workspace11/1, Scope13/1
  Body Sensor/2 -> Scope14/1, To Workspace10/1
  Body Sensor/3 -> Scope12/1, To Workspace12/1
  Body Sensor1/1 -> To Workspace14/1, Scope16/1
  Body Sensor1/2 -> Scope17/1, To Workspace13/1
  Body Sensor1/3 -> Scope15/1, To Workspace15/1
  Saturation/1 -> Add/2
  Ramp/1 -> Saturation/1
  Saturation1/1 -> Add1/2
  Ramp1/1 -> Saturation1/1
  connections:
  RootPart/RConn1 -- Weld/LConn1
  Weld/RConn1 -- pasador-1/LConn1
  L2-1/RConn1 -- Revolute/LConn1
  Revolute/RConn1 -- bloque1-1/LConn1
  L1-1/RConn1 -- Revolute1/LConn1
  Revolute1/RConn1 -- L2-1/LConn1
  bloque1-1/RConn2 -- Planar/LConn1
  Planar/RConn1 -- bloque-1/LConn1
  L2-2/RConn1 -- Revolute2/LConn1
  Revolute2/RConn1 -- bloque-1/LConn2
  pasador-1/RConn1 -- Planar1/LConn1
  Planar1/RConn1 -- bloque1-1/LConn2
  bloque1-1/RConn3 -- Revolute3/LConn1
  Revolute3/RConn1 -- L1-2/LConn1
  L1-2/RConn1 -- Revolute4/LConn1
  Revolute4/RConn1 -- L2-2/LConn1
  pasador-1/RConn2 -- Revolute5/LConn1
  Revolute5/RConn1 -- L1-1/LConn1
  RootGround/RConn1 -- Weld1/LConn1
  Weld1/RConn1 -- RootPart/LConn1
  RootGround/LConn1 -- Machine Environment/RConn1
  Joint Sensor/LConn1 -- Revolute5/RConn2
  Joint Actuator/RConn1 -- Revolute5/LConn2
  Joint Actuator1/RConn1 -- Revolute3/LConn2
  Joint Sensor1/LConn1 -- Revolute3/RConn2
  Body Sensor/LConn1 -- bloque1-1/RConn1
  Body Sensor1/LConn1 -- bloque-1/RConn1
